simulink library "microdaq_lib"  (R2024b)
settings: Solver=ode45  StartTime=0.0  StopTime=10.0  RelTol=1e-3
libraries: etargetslib x4
settings Model: Creator=bas  LastModifiedBy=benia
settings SolverCC: AlgebraicLoopSolver=TrustRegion
settings DataIOCC: LimitDataPoints=on  SaveFormat=Array  SignalLoggingSaveFormat=ModelDataLogs  ReturnWorkspaceOutputs=off
settings OptimizationCC: BlockReduction=off  BooleanDataType=off  LifeSpan=inf
settings DebuggingCC: SaveWithParameterizedLinksMsg=none  UnderspecifiedInitializationDetection=Classic  MergeDetectMultiDrivingBlocksExec=none  SignalResolutionControl=TryResolveAllWithWarning  MultiTaskDSMMsg=warning  MultiTaskCondExecSysMsg=none  UnconnectedInputMsg=warning  UnconnectedOutputMsg=warning  UnconnectedLineMsg=warning  StateNameClashWarn=warning  SFUnexpectedBacktrackingDiag=warning  SFNoUnconditionalDefaultTransitionDiag=warning  SFExecutionAtInitializationDiag=none  ArithmeticOperatorsInVariantConditions=warning
settings HardwareCC: ProdBitPerPointer=32  ProdBitPerSizeT=32  ProdBitPerPtrDiffT=32  ProdLargestAtomicFloat=None  ProdIntDivRoundTo=Undefined  ProdEndianess=Unspecified  ProdWordSize=32  ProdHWDeviceType=32-bit Generic  TargetUnknown=on
settings ModelReferenceCC: PropagateSignalLabelsOutOfModel=off
settings SFSimCC: SimUseLocalCustomCode=off  CustomCodeUndefinedFunction=UseInterfaceOnly
settings RTWCC: RTWUseLocalCustomCode=off  GPUComputeCapability=3.5
settings CodeAppCC: StateflowObjectComments=on
settings GRTTargetCC: TargetLangStandard=C89/C90 (ANSI)
settings ConfigComp: CovMetricSettings=dw  CovSaveCumulativeToWorkspaceVar=on  CovSaveSingleToWorkspaceVar=on  CovExternalEMLEnable=off

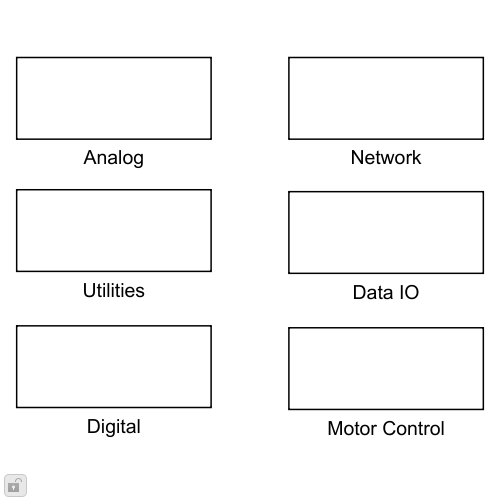
[thumbnail: Simulink's stored preview of the top-level diagram]
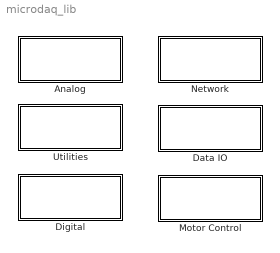
== system microdaq_lib ==
  Analog : Subsystem
  Data IO : Subsystem
  Digital : Subsystem
  Motor Control : Subsystem
  Network : Subsystem
  Utilities : Subsystem

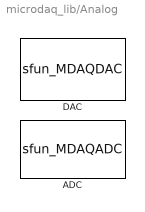
== system microdaq_lib/Analog ==
  ADC : S-Function  FunctionName=sfun_MDAQADC  Parameters=pChannel, pChannelCount, pRange, pMode, pAveraging, SampleTime  SFunctionDeploymentMode=off  EnableBusSupport=off  mask(ADC block){pChannel=[ 1 ], pChannelCount=ones([1 1 ]), pRange=[-10, 10], pMode=0, pAveraging=Off, SampleTime=-1}
      mask prompts: pChannel "Channels:"; pChannelCount "P2:"; pRange "Range:"; pMode "Mode:"; pAveraging "Averaging:"; SampleTime "Sample time (-1 for inherited):"
      mask help:
      | This block reads MicroDAQ analog inputs (AI). Block detects
      | MicroDAQ analog inputs type and allows channel, range
      | and measurement type selection.
      | In order to select analog input channels scalar or vector
      | containing channel number have to be provided.
      | Input range can be selected by providing scalar or vector
      | with range identifiers. If single range provided it will
      | be applied for all selected channels.
      | Single-ended or differential measurement type can be selected.
      | Scalar or vector with 1 and 0 values can be provided to enable
      | and disable differential mode.
      | If scalar is provided it will be applied for all used channels
      |
      | Averaging allows to increase measurement accuracy by calculating
      | average from 4-256 ADC samples.
      mask init:
      | if size(pChannel, 1) > 1 
      |     error('Wrong channel - scalar or single row vector expected');
      | end
      | 
      | if size(pMode, 1) > 1 
      |     error('Wrong channel - scalar or single row vector expected');
      | end
      | 
      | if size(pRange, 2) ~= 2
      |     error('Wrong range - matrix range [low,high;low,high;...] expected');
      | end
      | 
      | chCount = size(pChannel,2);
      | pChannelCount = chCount;
      | 
      | aiRangeSize = size(pRange, 1);
      | if aiRangeSize ~= 1 && aiRangeSize ~= chCount
      |     error('Range vector should match selected channels!')
      | end
      | 
      | aiModeSize = size(pMode, 1);
      | if aiModeSize ~= 1 && aiModeSize ~= chCount
      |     error('Range vector should match selected channels!')
      | end
      | 
      | if aiRangeSize == 1 
      |     range_tmp = pRange;
      |     pRange = ones(chCount,2);
      |     pRange(:,1) = range_tmp(1);
      |     pRange(:,2) = range_tmp(2);
      |     clear range_tmp;
      | end
      | 
      | if aiModeSize == 1
      |     pMode = ones(1,chCount) * pMode; 
      | end
      | 
      | pAveraging = pAveraging -1;
      | pRange = reshape(pRange', 1, chCount*2);
      | 
      | %result = mdaqCheckAdcParams(pChannel, pRange, pMode);
      | result = '';
      | if ~isempty(result)
      |     error(result);
      | end
      mask Help: <p>This block reads MicroDAQ analog inputs. Block supports different types of MicroDAQ analog inputs. In order to read more then one ADC channel provide array of channels to read in block 'Channels' parameter. Depending on 'Range' and 'Polarity' analog input range can be selected.</p>
      mask TypeOptions pAveraging: Off | x4 | x16 | x64 | x256
      mask Display:
      | color('blue');
      | text(0.05, 0.12, 'MicroDAQ', 'horizontalalignment', 'left');
      | color('black');
      | fprintf('\nADC\n\n\n\n');
      | color('gray');
      | 
      | 
      | fprintf('\n\nCH: %s\n\n', num2str(pChannel));
      | port_label('output',1,'Volt');
  DAC : S-Function  FunctionName=sfun_MDAQDAC  Parameters=pChannel, chCount, pRange, pInitValue, pTermValue, pUseInitTerm, SampleTime  SFunctionDeploymentMode=off  EnableBusSupport=off  mask(DAC block){pChannel=[ 1 ], pChannelCount=ones([1 1 ]), pRange=[0 5], pInitValue=0, pTermValue=0, pUseInitTerm=2, SampleTime=-1}
      mask prompts: pChannel "Channels:"; pChannelCount "P2:"; pRange "Range"; pInitValue "Initial value:"; pTermValue "Termination value:"; pUseInitTerm "Use Init/Term"; SampleTime "Sample time (-1 for inherited):"
      mask help:
      | This block writes data to MicroDAQ analog output module (AO).
      | Block detects MicroDAQ analog output type and allows
      | setting output range, initial and termination voltage.
      | The Range value can be a scalar or a vector that must
      | be the same length as the channel vector. If scalar value
      | is specified, that setting is replicated over the channel vector.
      | Different ranges can be set for each channel if ADC supports
      | more then one output range.
      | The Initial and Termination property can be a scalar or a vector
      |
      | Use Init/Term parameter allows to enable or disable setting
      | initial or/and termination voltage values. User can provide
      | scalar or vector with following values:
      | 0 - Initial and termination voltage value is ignored
      | 1 - Initial voltage value is used
      | 2 - Termination voltage value is used
      | 3 - Initial and termination voltage value is used
      mask init:
      | if size(pChannel, 1) > 1 
      |     error('Wrong channel - scalar or single row vector expected');
      | end
      | 
      | if size(pRange, 2) ~= 2
      |     error('Wrong range - matrix range [low,high;low,high;...] expected');
      | end
      | 
      | chCount = size(pChannel,2);
      | pChannelCount = chCount;
      | 
      | aoRangeSize = size(pRange, 1);
      | if aoRangeSize ~= 1 && aoRangeSize ~= chCount
      |     error('Range vector should match selected AI channels!')
      | end
      | 
      | if size(pInitValue,1) > 1
      |     error('Wrong initial value - scalar or single row vector expected')
      | end
      | 
      | if size(pTermValue,1) > 1
      |     error('Wrong termination value - scalar or single row vector expected')
      | end
      | 
      | if size(pUseInitTerm,1) > 1
      |     error('Wrong use init/term value - scalar or single row vector expected')
      | end
      | 
      | if chCount ~= size(pInitValue,2) &&  size(pInitValue,2) ~= 1
      |     error('Initial value vector should match selected AI channels!')
      | end
      | 
      | if chCount ~= size(pTermValue,2) &&  size(pTermValue,2) ~= 1
      |     error('Termination value vector should match selected AI channels!')
      | end
      | 
      | if chCount ~= size(pUseInitTerm,2) &&  size(pUseInitTerm,2) ~= 1
      |     error('Use init/term vector should match selected AI channels!')
      | end
      | 
      | if aoRangeSize == 1 
      |     range_tmp = pRange;
      |     pRange = ones(chCount,2);
      |     pRange(:,1) = range_tmp(1);
      |     pRange(:,2) = range_tmp(2);
      |     clear range_tmp;
      | end
      | 
      | pRange = reshape(pRange', 1, chCount*2);
      | 
      | if  size(pInitValue,2) == 1
      |     pInitValue = ones(1,chCount) * pInitValue;
      | end
      | 
      | if  size(pTermValue,2) == 1
      |     pTermValue = ones(1,chCount) * pTermValue;
      | end
      | 
      | if  size(pUseInitTerm,2) == 1
      |     pUseInitTerm = ones(1,chCount) * pUseInitTerm;
      | end
      | 
      | %result = mdaqCheckDacParams(pChannel, pRange);
      | result = '';
      | if ~isempty(result)
      |     error(result);
      | end
      mask Help: <p>This block was generated automatically by the Legacy Code Tool. For detailed help on this tool, call<a href="matlab:legacy_code('help')"> legacy_code('help')</a>.</p>
      mask Display:
      | color('blue');
      | text(0.98, 0.12, 'MicroDAQ', 'horizontalalignment', 'right');
      | color('black');
      | fprintf('\nDAC\n\n\n\n');
      | color('gray');
      | fprintf('\nCH: %s\n',num2str(pChannel));
      | port_label('input',1,'Volt');

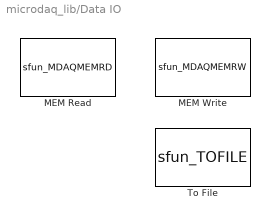
== system microdaq_lib/Data IO ==
  "MEM Read " : S-Function  FunctionName=sfun_MDAQMEMRD  Parameters=pMemAddr, pArraySize, pVectorSize, pPeriodic, SampleTime  SFunctionDeploymentMode=off  EnableBusSupport=off  mask(Read memory block){pMemAddr=1, pArraySize=1, pVectorSize=1, Periodic=on, SampleTime=-1}
      mask prompts: pMemAddr "Start index:"; pArraySize "Size:"; pVectorSize "Vector size:"; Periodic "Circular memory buffer"; SampleTime "Sample time (-1 for inherited):"
      mask help:
      | This block reads data from MicroDAQ memory. Block with mdaq_mem_write function can be used to change Standalone model parameters.
      |
      | 'Size' parameter defines memory size used by block, e.g in order to read 1 sample of vector of size 4 user needs to set 'Size' parameter to 4 and 'Vector size' to 4.
      mask init:
      | if (Periodic)
      |     pPeriodic = 1;
      | else
      |     pPeriodic = 0;
      | end
      | 
      | pMemAddr = pMemAddr - 1;
      mask Display:
      | color('blue');
      | text(0.98, 0.13, 'MicroDAQ', 'horizontalalignment', 'right');
      | color('black');
      | fprintf('MEM Read\n\n\n');
      | color('gray');
  "MEM Write  " : S-Function  FunctionName=sfun_MDAQMEMRW  Parameters=pMemAddr, pArraySize, pVectorSize, pOverwrite, SampleTime  SFunctionDeploymentMode=off  EnableBusSupport=off  mask(Write Memory block){pMemAddr=1, pArraySize=1, pVectorSize=1, Overwrite=on, SampleTime=-1}
      mask prompts: pMemAddr "Index:"; pArraySize "Size:"; pVectorSize "Vector size:"; Overwrite "Circular buffer"; SampleTime "Sample time (-1 for inherited):"
      mask help:
      | This block writes data to MicroDAQ memory. Block with mdaq_mem_read function can be used to get data from Standalone model.
      |
      | 'Size' parameter defines memory size used by block, e.g in order to write 100 samples of vector of size 4 user needs to set 'Size' parameter to 400 and 'Vector size' to 4.
      mask init:
      | if (Overwrite)
      |     pOverwrite  = 1; 
      | else
      |     pOverwrite  = 0; 
      | end
      | pMemAddr = pMemAddr - 1;
      | 
      | pArraySize = pArraySize * pVectorSize;
      mask Display:
      | color('blue');
      | text(0.98, 0.13, 'MicroDAQ', 'horizontalalignment', 'right');
      | color('black');
      | fprintf('MEM Write\n\n\n');
      | color('gray');
  To File : S-Function  FunctionName=sfun_TOFILE  Parameters=pFileName, pMode, pBufSize, pVecSize, pType, SampleTime  SFunctionDeploymentMode=off  EnableBusSupport=off  mask(To File){pName='data.txt', pType=Text, pMode=Create, pBufSize=10, pVecSize=1, SampleTime=-1}
      mask prompts: pName "File name:"; pType "Filt type:"; pMode "Mode:"; pBufSize "Vector buffer size:"; pVecSize "Vector size:"; SampleTime "Sample time (-1 for inherited):"
      mask help:
      | This block writes data to file. Files are created on user disk in 'dsp/data' directory. Files can be downloaded via web browser or mass storage interface.
      | Data can be written to file in text of binary format, data can be appended to previous content of the file or file content can be truncated. To avoid time time consuming wirte operation during every simulation step block can buffer data.
      mask init:
      | pFileName = [int8(pName),0];
      | pBufSize = 10;
      mask Help: <p>This block was generated automatically by the Legacy Code Tool. For detailed help on this tool, call<a href="matlab:legacy_code('help')"> legacy_code('help')</a>.</p>
      mask TypeOptions pType: Text | Binary
      mask TypeOptions pMode: Create | Append
      mask Display:
      | color('blue');
      | text(0.98, 0.13, 'MicroDAQ', 'horizontalalignment', 'right');
      | color('black');
      | fprintf('To File\n\n\n');
      | color('gray');
      | fprintf(pName);

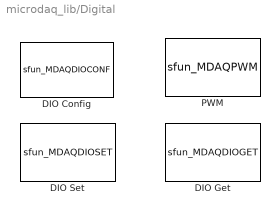
== system microdaq_lib/Digital ==
  DIO Config : S-Function  FunctionName=sfun_MDAQDIOCONF  Parameters=SParameter1, SParameter2, SParameter3, SParameter4, SParameter5, SParameter6, SParameter7, SParameter8, SParameter9, SParameter10  SFunctionDeploymentMode=off  EnableBusSupport=off  mask(DIO Config){SParameter1=Enable, SParameter2=Enable, SParameter3=Enable, SParameter4=Enable, SParameter5=Enable, SParameter6=Enable, SParameter7=Input, SParameter8=Output, SParameter9=Output, SParameter10=Input}
      mask prompts: SParameter1 "ENC1:"; SParameter2 "ENC2:"; SParameter3 "PWM1:"; SParameter4 "PWM2:"; SParameter5 "PWM3:"; SParameter6 "UART:"; SParameter7 "DIO1...8 direction:"; SParameter8 "DIO9...16 direction:"; SParameter9 "DIO17...24 direction:"; SParameter10 "DIO25...32 direction:"
      mask help: This block configures DIO alternative functions and DIO direction.
      mask init:
      | SParameter1 = SParameter1 - 1;
      | SParameter2 = SParameter2 - 1;
      | SParameter3 = SParameter3 - 1;
      | SParameter4 = SParameter4 - 1;
      | SParameter5 = SParameter5 - 1;
      | SParameter6 = SParameter6 - 1;
      | SParameter7 = SParameter7 - 1;
      | SParameter8 = SParameter8 - 1;
      | SParameter9 = SParameter9 - 1;
      | SParameter10 = SParameter10 - 1;
      mask TypeOptions SParameter1: Disable | Enable
      mask TypeOptions SParameter2: Disable | Enable
      mask TypeOptions SParameter3: Disable | Enable
      mask TypeOptions SParameter4: Disable | Enable
      mask TypeOptions SParameter5: Disable | Enable
      mask TypeOptions SParameter6: Disable | Enable
      mask TypeOptions SParameter7: Output | Input
      mask TypeOptions SParameter8: Output | Input
      mask TypeOptions SParameter9: Output | Input
      mask TypeOptions SParameter10: Output | Input
      mask Display:
      | color('blue');
      | text(0.98, 0.13, 'MicroDAQ', 'horizontalalignment', 'right');
      | color('black');
      | fprintf('DIO Config\n\n');
  DIO Get : S-Function  FunctionName=sfun_MDAQDIOGET  Parameters=pDIOpin, SampleTime  SFunctionDeploymentMode=off  EnableBusSupport=off  mask(DIO Get){pDIOpin=DIO1, SampleTime=-1}
      mask prompts: pDIOpin "DIO pin:"; SampleTime "Sample time (-1 for inherited):"
      mask help: This block reads MicroDAQ DIO input state.
      mask TypeOptions pDIOpin: DIO1 | DIO2 | DIO3 | DIO4 | DIO5 | DIO6 | DIO7 | DIO8 | DIO9 | DIO10 | DIO11 | DIO12 | DIO13 | DIO14 | DIO15 | DIO16 | DIO17 | DIO18 | DIO19 | DIO20 | DIO21 | DIO22 | DIO23 | DIO24 | DIO25 | DIO26 | DIO27 | DIO28 | DIO29 | DIO30 | DIO31 | DIO32
      mask Display:
      | color('blue');
      | text(0.98, 0.13, 'MicroDAQ', 'horizontalalignment', 'right');
      | color('black');
      | fprintf('DIO Get\n\n');
      | color('gray');
      | fprintf('\nDIO%d',pDIOpin);
  DIO Set : S-Function  FunctionName=sfun_MDAQDIOSET  Parameters=pDIOpin, pDIOdir, pDIOinitValue, pDIOtermValue SampleTime  SFunctionDeploymentMode=off  EnableBusSupport=off  mask(DIO Set){pDIOpin=DIO1, pDIOdir=ones([1 1 ]), pDIOinitValue=Low, pDIOtermValue=Low, SampleTime=-1}
      mask prompts: pDIOpin "DIO pin number:"; pDIOdir "Direction:"; pDIOinitValue "DIO init value:"; pDIOtermValue "DIO term value:"; SampleTime "Sample time (-1 for inherited):"
      mask help: This block sets MicroDAQ DIO state.
      mask init:
      | pDIOdir = 0;
      mask TypeOptions pDIOpin: DIO1 | DIO2 | DIO3 | DIO4 | DIO5 | DIO6 | DIO7 | DIO8 | DIO9 | DIO10 | DIO11 | DIO12 | DIO13 | DIO14 | DIO15 | DIO16 | DIO17 | DIO18 | DIO19 | DIO20 | DIO21 | DIO22 | DIO23 | DIO24 | DIO25 | DIO26 | DIO27 | DIO28 | DIO29 | DIO30 | DIO31 | DIO32
      mask TypeOptions pDIOinitValue: High | Low
      mask TypeOptions pDIOtermValue: High | Low
      mask Display:
      | color('blue');
      | text(0.98, 0.13, 'MicroDAQ', 'horizontalalignment', 'right');
      | color('black');
      | fprintf('DIO Set\n\n');
      | color('gray');
      | fprintf('\nDIO%d',pDIOpin);
  PWM : S-Function  FunctionName=sfun_MDAQPWM  Parameters=pModule, pPeriod, pPolarity, SampleTime  SFunctionDeploymentMode=off  EnableBusSupport=off  mask(PWM block){pModule=PWM1, pPeriod=1000, pPolarity=Active HIGH, SampleTime=-1}
      mask prompts: pModule "PWM module:"; pPeriod "Period [us]:"; pPolarity "Polarity:"; SampleTime "Sample time (-1 for inherited):"
      mask help:
      | This block sets MicroDAQ PWM outputs. Block controls one PWM module which contains A and B channels.
      | User can set PWM period in microseconds and select polarity of PWM waveform.
      | Block has two inputs A and B, when PWM block is configured to work with constant PERIOD input range is 0 - 100% .
      mask init:
      | pPolarity = pPolarity -1;
      mask TypeOptions pModule: PWM1 | PWM2 | PWM3
      mask TypeOptions pPolarity: Active HIGH | Active LOW
      mask Display:
      | color('blue');
      | text(0.98, 0.13, 'MicroDAQ', 'horizontalalignment', 'right');
      | color('black');
      | fprintf('PWM\n\n');
      | color('gray');
      | fprintf('\nPWM%d',pModule);
      | color('black');
      | port_label('input',1,'A');
      | port_label('input',2,'B');

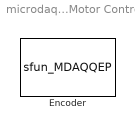
== system microdaq_lib/Motor Control ==
  Encoder : S-Function  FunctionName=sfun_MDAQQEP  Parameters=pChannel, SampleTime  SFunctionDeploymentMode=off  EnableBusSupport=off  mask(Encoder block){pChannel=ENC1, SampleTime=0}
      mask prompts: pChannel "Module:"; SampleTime "Sample time (-1 for inherited):"
      mask help: This block reads MicroDAQ quadrature encoder inputs (ENC).
      mask TypeOptions pChannel: ENC1 | ENC2
      mask Display:
      | color('blue');
      | text(0.05, 0.13, 'MicroDAQ', 'horizontalalignment', 'left');
      | color('black');
      | fprintf('Encoder\n\n');
      | color('gray');
      | fprintf('\nCH%d',pChannel);
      | color('black');
      | port_label('output',1,'Pos');
      | port_label('output',2,'Dir');
      | port_label('input',1,'Reset');

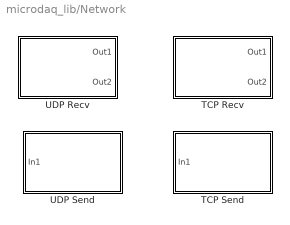
== system microdaq_lib/Network ==
  TCP Recv : Subsystem  mask(TCP/IP Recv){IPAddrStr='10.10.1.10', Port=5000, Blocking=off, Timeout=250, Datatype=double, SizePack=1, SampleTime=-1}
      mask prompts: IPAddrStr "Remote IP address:"; Port "Remote port:"; Timeout "Timeout (ms):"; Datatype "Data type:"; SizePack "Message size (in data type units):"; SampleTime "Sample time:"
      mask help: Receive TCP/IP packets from given IP port and address.
      mask init:
      | % Convert string IP Address to bytes
      | % for use in S-function
      | IPAddr = double(IPAddrStr);
      | % TCP Protocol
      | Protocol = 0;
      | % Construct data type expression for Pack block
      | %packdt = repmat({Datatype},SizePack,1);
      | packdt = {Datatype};
      | % Any better way to find data type size?
      | eval(['dummy = ',Datatype,'(0);']);
      | dummy = whos('dummy');
      | Size = SizePack*dummy.bytes;
      mask TypeOptions Datatype: double | single | uint8 | uint16 | uint32 | int8 | int16 | int32 | boolean
      mask Display:
      | color('blue');
      | text(0.98, 0.13, 'MicroDAQ', 'horizontalalignment', 'right');
      | color('black');
      | fprintf('TCP/IP Recv\n\n\n');
      | color('gray');
  TCP Send : Subsystem  mask(TCP/IP Send){IPAddrStr='10.10.1.10', Port=5000, Blocking=off, Timeout=250, Datatype=double, SizePack=1, SampleTime=-1}
      mask prompts: IPAddrStr "Remote IP address:"; Port "Remote port:"; Timeout "Timeout (ms):"; Datatype "Data type:"; SizePack "Message size (in data type units):"; SampleTime "Sample time:"
      mask help: Send TCP/IP packets to given IP port and address.
      mask init: same as microdaq_lib/Network/TCP Recv
      mask TypeOptions Datatype: double | single | uint8 | uint16 | uint32 | int8 | int16 | int32 | boolean
      mask Display:
      | color('blue');
      | text(0.98, 0.13, 'MicroDAQ', 'horizontalalignment', 'right');
      | color('black');
      | fprintf('TCP/IP Send\n\n\n');
      | color('gray');
  UDP Recv : Subsystem  mask(UDP Recv){IPAddrStr='10.10.1.10', Port=5001, Blocking=off, Timeout=250, Datatype=double, SizePack=1, SampleTime=-1}
      mask prompts: IPAddrStr "Remote IP address:"; Port "Remote port:"; Timeout "Timeout (ms):"; Datatype "Data type:"; SizePack "Message size (in data type units):"; SampleTime "Sample time:"
      mask help: Receive UDP packets from given IP port and address.
      mask init:
      | % Convert string IP Address to bytes
      | % for use in S-function
      | IPAddr = double(IPAddrStr);
      | % UDP Protocol
      | Protocol = 1;
      | % Construct data type expression for Pack block
      | %packdt = repmat({Datatype},SizePack,1);
      | packdt = {Datatype};
      | % Any better way to find data type size?
      | eval(['dummy = ',Datatype,'(0);']);
      | dummy = whos('dummy');
      | Size = SizePack*dummy.bytes;
      mask TypeOptions Datatype: double | single | uint8 | uint16 | uint32 | int8 | int16 | int32 | boolean
      mask Display:
      | color('blue');
      | text(0.98, 0.13, 'MicroDAQ', 'horizontalalignment', 'right');
      | color('black');
      | fprintf('UDP Recv\n\n\n');
      | color('gray');
  UDP Send : Subsystem  mask(UDP Send){IPAddrStr='10.10.1.10', Port=5000, Blocking=off, Timeout=250, Datatype=double, SizePack=1, SampleTime=-1}
      mask prompts: IPAddrStr "Remote IP address:"; Port "Remote port:"; Timeout "Timeout (ms):"; Datatype "Data type:"; SizePack "Message size (in data type units):"; SampleTime "Sample time:"
      mask help: Send UDP packets to given IP port and address.
      mask init: same as microdaq_lib/Network/UDP Recv
      mask TypeOptions Datatype: double | single | uint8 | uint16 | uint32 | int8 | int16 | int32 | boolean
      mask Display:
      | color('blue');
      | text(0.98, 0.13, 'MicroDAQ', 'horizontalalignment', 'right');
      | color('black');
      | fprintf('UDP Send\n\n\n');
      | color('gray');

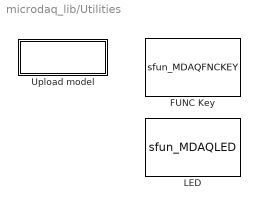
== system microdaq_lib/Utilities ==
  FUNC Key : S-Function  FunctionName=sfun_MDAQFNCKEY  Parameters=pDIOFuncKey, SampleTime  SFunctionDeploymentMode=off  EnableBusSupport=off  mask(FUNC Key){pDIOFuncKey=F1, SampleTime=-1}
      mask prompts: pDIOFuncKey "Function key:"; SampleTime "Sample time (-1 for inherited):"
      mask help: This block allows you to read MicroDAQ function key state (F1/F2).
      mask Help: <p>This block was generated automatically by the Legacy Code Tool. For detailed help on this tool, call<a href="matlab:legacy_code('help')"> legacy_code('help')</a>.</p>
      mask TypeOptions pDIOFuncKey: F1 | F2
      mask Display:
      | color('blue');
      | text(0.98, 0.13, 'MicroDAQ', 'horizontalalignment', 'right');
      | color('black');
      | fprintf('FUNC Key\n\n');
      | color('gray');
      | fprintf('\nF%d',pDIOFuncKey);
  LED : S-Function  FunctionName=sfun_MDAQLED  Parameters=SParameter1  SFunctionDeploymentMode=off  EnableBusSupport=off  mask(LED){SParameter1=D1}
      mask prompts: SParameter1 "Choose LED:"
      mask help:
      | This block allows you to control the built-in LEDs of MicroDAQ.
      | Setting input to 1 will switch on the selected LED.
      mask TypeOptions SParameter1: D1 | D2
      mask Display:
      | color('blue');
      | text(0.98, 0.13, 'MicroDAQ', 'horizontalalignment', 'right');
      | color('black');
      | fprintf('LED\n\n');
      | color('gray');
      | fprintf('\nD%d',SParameter1);
  Upload model : Subsystem  mask(UPLOAD block){ShowInLibBrowser=on}
      mask help:
      | This block saves DSP application on target in non-volatile memory.
      | After MicroDAQ power up DSP application will start automatically.
      | In order to upload DSP application load model on target and than double
      | click on UPLOAD block.
      |
      | DSP application will be placed on user disk in directory 'dsp'. In order to
      | turn of autostart of DSP application connect MicroDAQ with USB cable and
      | delete 'dsp-firmware.out' file in 'dsp' directory.
      settings: OpenFcn=mlink_download('', getpref('microdaq','TargetRoot'), 1)
      mask Display: disp( 'UPLOAD' )

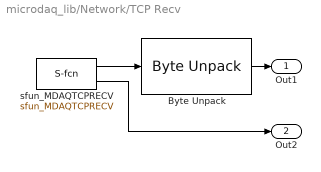
== system microdaq_lib/Network/TCP Recv ==
  Byte Unpack : etargetslib/Byte Unpack  dimensions={[1]}  datatypes={'double'}  byteAlign=1
  sfun_MDAQTCPRECV : S-Function  FunctionName=sfun_MDAQTCPRECV  Parameters=IPAddr, Port, Blocking, Timeout, Protocol, Size, SampleTime  SFunctionDeploymentMode=off  EnableBusSupport=off
  Out1 : Outport
  Out2 : Outport  Port=2
  wires:
  sfun_MDAQTCPRECV/1 -> Byte Unpack/1
  sfun_MDAQTCPRECV/2 -> Out2/1
  Byte Unpack/1 -> Out1/1

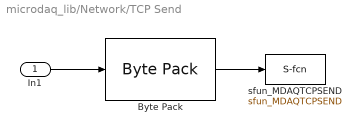
== system microdaq_lib/Network/TCP Send ==
  In1 : Inport  PortDimensions=SizePack
  Byte Pack : etargetslib/Byte Pack  datatypes={'double'}  byteAlign=1
  sfun_MDAQTCPSEND : S-Function  FunctionName=sfun_MDAQTCPSEND  Parameters=IPAddr, Port, Blocking, Timeout, Protocol, Size, SampleTime  SFunctionDeploymentMode=off  EnableBusSupport=off
  wires:
  In1/1 -> Byte Pack/1
  Byte Pack/1 -> sfun_MDAQTCPSEND/1

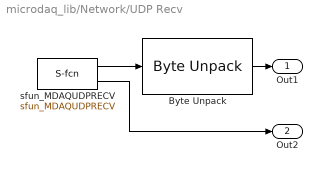
== system microdaq_lib/Network/UDP Recv ==
  Byte Unpack : etargetslib/Byte Unpack  dimensions={[1]}  datatypes={'double'}  byteAlign=1
  sfun_MDAQUDPRECV : S-Function  FunctionName=sfun_MDAQUDPRECV  Parameters=IPAddr, Port, Blocking, Timeout, Protocol, Size, SampleTime  SFunctionDeploymentMode=off  EnableBusSupport=off
  Out1 : Outport
  Out2 : Outport  Port=2
  wires:
  Byte Unpack/1 -> Out1/1
  sfun_MDAQUDPRECV/2 -> Out2/1
  sfun_MDAQUDPRECV/1 -> Byte Unpack/1

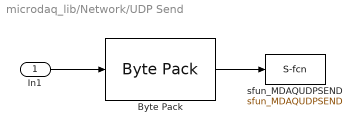
== system microdaq_lib/Network/UDP Send ==
  In1 : Inport  PortDimensions=SizePack
  Byte Pack : etargetslib/Byte Pack  datatypes={'double'}  byteAlign=1
  sfun_MDAQUDPSEND : S-Function  FunctionName=sfun_MDAQUDPSEND  Parameters=IPAddr, Port, Blocking, Timeout, Protocol, Size, SampleTime  SFunctionDeploymentMode=off  EnableBusSupport=off
  wires:
  In1/1 -> Byte Pack/1
  Byte Pack/1 -> sfun_MDAQUDPSEND/1

== system microdaq_lib/Utilities/Upload model ==
  note: This block saves DSP application on target in non-volatile memory.
      | After MicroDAQ power up DSP application will start automatically.
      | In order to upload DSP application load model on target and than double
      | click on UPLOAD block.
      |
      | DSP application will be placed on user disk in directory 'dsp'. In order to
      | turn of autostart of DSP application connect MicroDAQ with USB cable and
      | delete 'dsp-firmware.out' file in 'dsp' directory.
  note: Saves DSP model on MicroDAQ
